simulink model "simpleThermalModel_old"  (R2022a)
settings: Solver=VariableStepAuto  StartTime=0.0  StopTime=36000  RelTol=1e-3
undefined symbols (not defined in the file): param
libraries: fl_lib x53, nesl_utility x15
settings Model: Creator=BrunoMattos  LastModifiedBy=BrunoMattos

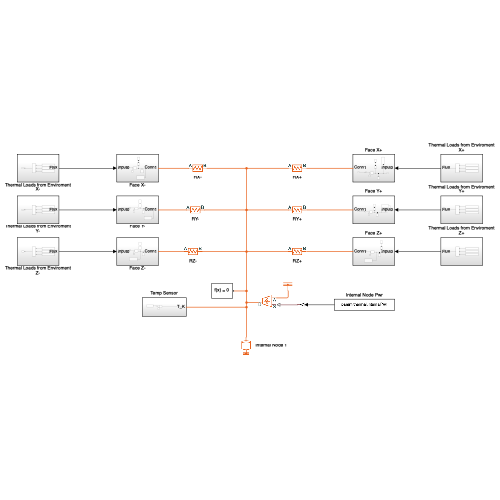
[thumbnail: Simulink's stored preview of the top-level diagram]
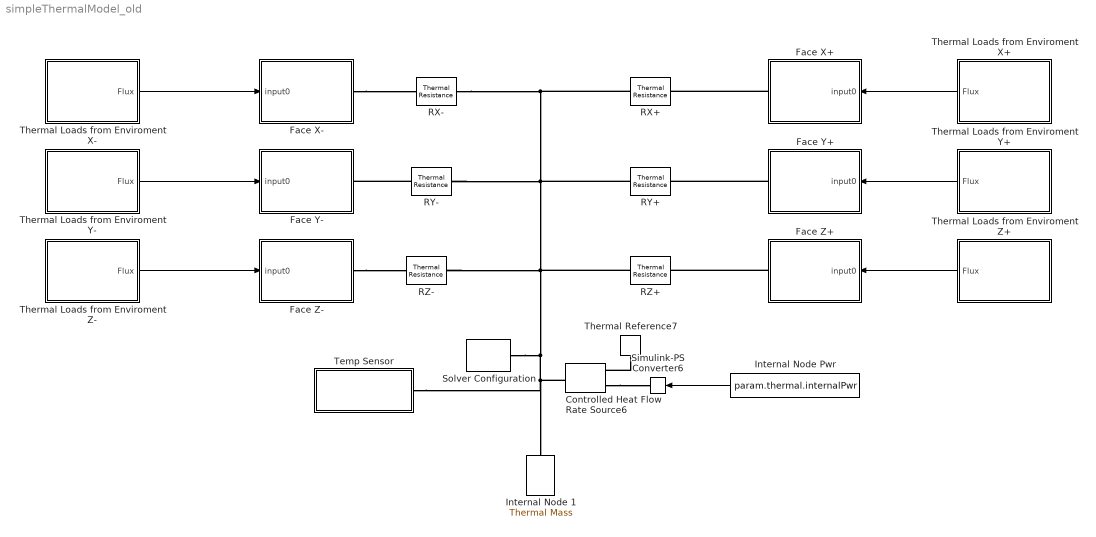
== system simpleThermalModel_old ==
  Controlled Heat Flow Rate Source6 : fl_lib/Thermal/Thermal Sources/Controlled Heat Flow Rate Source
      settings: SourceProductBaseCode=PW,SS,VE
  Face X+ : Subsystem
  Face X- : Subsystem
  Face Y+ : Subsystem
  Face Y- : Subsystem
  Face Z+ : Subsystem
  Face Z- : Subsystem
  Internal Node 1 : fl_lib/Thermal/Thermal Elements/Thermal Mass  mass=param.internalNodeMass(1) kg  sp_heat=param.internalNodeCp(1) J/(K*kg)  T_specify=off  T_priority=High  T=300 K  T_nominal_specify=off  T_nominal_unit=K  T_nominal_value=1  Q_specify=off  Q_priority=None  Q=0 W  Q_nominal_specify=off  Q_nominal_unit=W  Q_nominal_value=1
      settings: SourceProductBaseCode=PW,SS,VE
  Internal Node Pwr : FromWorkspace  VariableName=param.thermal.internalPwr
  RX+ : fl_lib/Thermal/Thermal Elements/Thermal Resistance  resistance=param.resistance(1) K/W  T_specify=off  T_priority=None  T=0 K  T_nominal_specify=off  T_nominal_unit=K  T_nominal_value=1  Q_specify=off  Q_priority=None  Q=0 W  Q_nominal_specify=off  Q_nominal_unit=W  Q_nominal_value=1
      settings: SourceProductBaseCode=PW,SS,VE
  RX- : fl_lib/Thermal/Thermal Elements/Thermal Resistance  resistance=param.resistance(2) K/W  T_specify=off  T_priority=None  T=0 K  T_nominal_specify=off  T_nominal_unit=K  T_nominal_value=1  Q_specify=off  Q_priority=None  Q=0 W  Q_nominal_specify=off  Q_nominal_unit=W  Q_nominal_value=1
      settings: SourceProductBaseCode=PW,SS,VE
  RY+ : fl_lib/Thermal/Thermal Elements/Thermal Resistance  resistance=param.resistance(3) K/W  T_specify=off  T_priority=None  T=0 K  T_nominal_specify=off  T_nominal_unit=K  T_nominal_value=1  Q_specify=off  Q_priority=None  Q=0 W  Q_nominal_specify=off  Q_nominal_unit=W  Q_nominal_value=1
      settings: SourceProductBaseCode=PW,SS,VE
  RY- : fl_lib/Thermal/Thermal Elements/Thermal Resistance  resistance=param.resistance(4) K/W  T_specify=off  T_priority=None  T=0 K  T_nominal_specify=off  T_nominal_unit=K  T_nominal_value=1  Q_specify=off  Q_priority=None  Q=0 W  Q_nominal_specify=off  Q_nominal_unit=W  Q_nominal_value=1
      settings: SourceProductBaseCode=PW,SS,VE
  RZ+ : fl_lib/Thermal/Thermal Elements/Thermal Resistance  resistance=param.resistance(5) K/W  T_specify=off  T_priority=None  T=0 K  T_nominal_specify=off  T_nominal_unit=K  T_nominal_value=1  Q_specify=off  Q_priority=None  Q=0 W  Q_nominal_specify=off  Q_nominal_unit=W  Q_nominal_value=1
      settings: SourceProductBaseCode=PW,SS,VE
  RZ- : fl_lib/Thermal/Thermal Elements/Thermal Resistance  resistance=param.resistance(6) K/W  T_specify=off  T_priority=None  T=0 K  T_nominal_specify=off  T_nominal_unit=K  T_nominal_value=1  Q_specify=off  Q_priority=None  Q=0 W  Q_nominal_specify=off  Q_nominal_unit=W  Q_nominal_value=1
      settings: SourceProductBaseCode=PW,SS,VE
  Simulink-PS Converter6 : nesl_utility/Simulink-PS Converter  PhysicalDomain=network_engine_domain  SubClassName=ps_input  LeftPortType=input  RightPortType=output  PseudoPeriodic=off  Frequencies=[]  NoiseDistribution=none  NoiseParameters=[]  Unit=1  AffineConversion=off  FilteringAndDerivatives=provide  SimscapeFilterOrder=1  InputFilterTimeConstant=0.001  UdotUserProvided=0
      settings: SourceProductBaseCode=SS,PW,VE
  Solver Configuration : nesl_utility/Solver Configuration  PhysicalDomain=network_engine_domain  SubClassName=solver  LeftPortType=input  RightPortType=generic  Tones=[]  Harmonics=[]  SimulateNoise=off  Profile=off  UseLocalSampling=off  EnableSwitchedLinearOptims=on  FrequencyDomain=off  UseCCode=off  RelTol=0.001  AbsTol=0.001  MinStep=1e-09  ToWorkspace=off  RevertToSquareIcSolve=off  NumHomotopyIterations=100  PhasorMode=off  PhasorModeNumHarmonics=1  IndexReductionMethod=DerivativeReplacement  DoDC=off  ResidualTolerance=1e-09  UseLocalSolver=off  LocalSolverChoice=NE_BACKWARD_EULER_ADVANCER  LocalSolverSampleTime=0.001  DoFixedCost=off  MaxNonlinIter=3  MaxModeIter=2  ComputeImpulses=off  ImpulseIterations=2  LinearAlgebra=auto  LinearAlgebraNumThread=0  EquationFormulation=NE_TIME_EF  DelaysMemoryBudget=1024  AutomaticFiltering=on  FilteringTimeConstant=0.001  PartitionStorageMethod=AS_NEEDED  PartitionMemoryBudget=1024  PartitionMethod=ROBUST
      settings: SourceProductBaseCode=SS,PW,VE
  Temp Sensor : Subsystem
  Thermal Loads from Enviroment X+ : Subsystem
  Thermal Loads from Enviroment X- : Subsystem
  Thermal Loads from Enviroment Y+ : Subsystem
  Thermal Loads from Enviroment Y- : Subsystem
  Thermal Loads from Enviroment Z+ : Subsystem
  Thermal Loads from Enviroment Z- : Subsystem
  Thermal Reference7 : fl_lib/Thermal/Thermal Elements/Thermal Reference
      settings: SourceProductBaseCode=PW,SS,VE
  wires:
  Thermal Loads from Enviroment X+/1(Flux) -> Face X+/1(input0)
  Thermal Loads from Enviroment Y+/1(Flux) -> Face Y+/1(input0)
  Thermal Loads from Enviroment Z+/1(Flux) -> Face Z+/1(input0)
  Thermal Loads from Enviroment X-/1(Flux) -> Face X-/1(input0)
  Thermal Loads from Enviroment Y-/1(Flux) -> Face Y-/1(input0)
  Thermal Loads from Enviroment Z-/1(Flux) -> Face Z-/1(input0)
  Internal Node Pwr/1 -> Simulink-PS Converter6/1
  connections:
  RX+/LConn1 -- RX-/RConn1 -- Temp Sensor/LConn1 -- Internal Node 1/LConn1 -- Controlled Heat Flow Rate Source6/LConn1 -- Solver Configuration/RConn1 -- RZ-/RConn1 -- RZ+/LConn1 -- RY-/RConn1 -- RY+/LConn1
  Thermal Reference7/LConn1 -- Controlled Heat Flow Rate Source6/RConn2
  Controlled Heat Flow Rate Source6/RConn1 -- Simulink-PS Converter6/RConn1
  Face X-/RConn1 -- RX-/LConn1
  RY-/LConn1 -- Face Y-/RConn1
  Face Z-/RConn1 -- RZ-/LConn1
  Face X+/RConn1 -- RX+/RConn1
  Face Y+/RConn1 -- RY+/RConn1
  Face Z+/RConn1 -- RZ+/RConn1

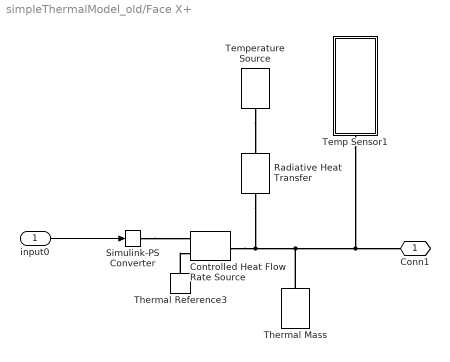
== system simpleThermalModel_old/Face X+ ==
  input0 : Inport
  Controlled Heat Flow Rate Source : fl_lib/Thermal/Thermal Sources/Controlled Heat Flow Rate Source
      settings: SourceProductBaseCode=PW,SS,VE
  Radiative Heat Transfer : fl_lib/Thermal/Thermal Elements/Radiative Heat Transfer  area=param.facesArea(1) m^2  rad_tr_coeff=param.krad(1) W/(K^4*m^2)  T_specify=off  T_priority=None  T=0 K  T_nominal_specify=off  T_nominal_unit=K  T_nominal_value=1  Q_specify=off  Q_priority=None  Q=0 W  Q_nominal_specify=off  Q_nominal_unit=W  Q_nominal_value=1
      settings: SourceProductBaseCode=PW,SS,VE  InternalSimscapePortConfiguration="{\"Bottom\":[],\"Left\":[{\"id\":\"A\",\"label\":\"A\",\"type\":\"foundation.thermal.thermal\"}],\"Right\":[{\"id\":\"B\",\"label\":\"B\",\"type\":\"foundation.thermal.thermal\"}],\"Top\":[]}"
  Simulink-PS Converter : nesl_utility/Simulink-PS Converter  PhysicalDomain=network_engine_domain  SubClassName=ps_input  LeftPortType=input  RightPortType=output  PseudoPeriodic=off  Frequencies=[]  NoiseDistribution=none  NoiseParameters=[]  Unit=1  AffineConversion=off  FilteringAndDerivatives=provide  SimscapeFilterOrder=1  InputFilterTimeConstant=0.001  UdotUserProvided=0
      settings: SourceProductBaseCode=SS,PW,VE
  Temp Sensor1 : Subsystem
  Temperature Source : fl_lib/Thermal/Thermal Sources/Temperature Source  temperature=7 K
      settings: SourceProductBaseCode=PW,SS,VE
  Thermal Mass : fl_lib/Thermal/Thermal Elements/Thermal Mass  mass=param.facesMass(1) kg  sp_heat=param.facesCp(1) J/(K*kg)  T_specify=off  T_priority=High  T=300 K  T_nominal_specify=off  T_nominal_unit=K  T_nominal_value=1  Q_specify=off  Q_priority=None  Q=0 W  Q_nominal_specify=off  Q_nominal_unit=W  Q_nominal_value=1
      settings: SourceProductBaseCode=PW,SS,VE
  Thermal Reference3 : fl_lib/Thermal/Thermal Elements/Thermal Reference
      settings: SourceProductBaseCode=PW,SS,VE
  Conn1 : PMIOPort  Side=Right
  wires:
  input0/1 -> Simulink-PS Converter/1
  connections:
  Simulink-PS Converter/RConn1 -- Controlled Heat Flow Rate Source/RConn1
  Thermal Reference3/LConn1 -- Controlled Heat Flow Rate Source/RConn2
  Temperature Source/LConn1 -- Radiative Heat Transfer/RConn1
  Radiative Heat Transfer/LConn1 -- Controlled Heat Flow Rate Source/LConn1 -- Thermal Mass/LConn1 -- Temp Sensor1/LConn1 -- Conn1/RConn1

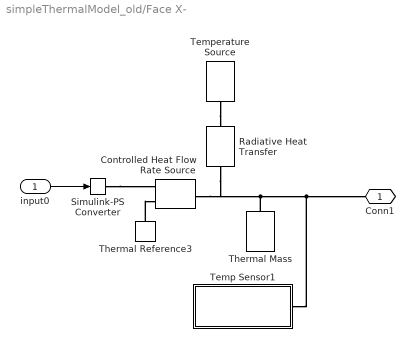
== system simpleThermalModel_old/Face X- ==
  input0 : Inport
  Controlled Heat Flow Rate Source : fl_lib/Thermal/Thermal Sources/Controlled Heat Flow Rate Source
      settings: SourceProductBaseCode=PW,SS,VE
  Radiative Heat Transfer : fl_lib/Thermal/Thermal Elements/Radiative Heat Transfer  area=param.facesArea(2) m^2  rad_tr_coeff=param.krad(2) W/(K^4*m^2)  T_specify=off  T_priority=None  T=0 K  T_nominal_specify=off  T_nominal_unit=K  T_nominal_value=1  Q_specify=off  Q_priority=None  Q=0 W  Q_nominal_specify=off  Q_nominal_unit=W  Q_nominal_value=1
      settings: SourceProductBaseCode=PW,SS,VE  InternalSimscapePortConfiguration="{\"Bottom\":[],\"Left\":[{\"id\":\"A\",\"label\":\"A\",\"type\":\"foundation.thermal.thermal\"}],\"Right\":[{\"id\":\"B\",\"label\":\"B\",\"type\":\"foundation.thermal.thermal\"}],\"Top\":[]}"
  Simulink-PS Converter : nesl_utility/Simulink-PS Converter  PhysicalDomain=network_engine_domain  SubClassName=ps_input  LeftPortType=input  RightPortType=output  PseudoPeriodic=off  Frequencies=[]  NoiseDistribution=none  NoiseParameters=[]  Unit=1  AffineConversion=off  FilteringAndDerivatives=provide  SimscapeFilterOrder=1  InputFilterTimeConstant=0.001  UdotUserProvided=0
      settings: SourceProductBaseCode=SS,PW,VE
  Temp Sensor1 : Subsystem
  Temperature Source : fl_lib/Thermal/Thermal Sources/Temperature Source  temperature=7 K
      settings: SourceProductBaseCode=PW,SS,VE
  Thermal Mass : fl_lib/Thermal/Thermal Elements/Thermal Mass  mass=param.facesMass(2) kg  sp_heat=param.facesCp(2) J/(K*kg)  T_specify=off  T_priority=High  T=300 K  T_nominal_specify=off  T_nominal_unit=K  T_nominal_value=1  Q_specify=off  Q_priority=None  Q=0 W  Q_nominal_specify=off  Q_nominal_unit=W  Q_nominal_value=1
      settings: SourceProductBaseCode=PW,SS,VE
  Thermal Reference3 : fl_lib/Thermal/Thermal Elements/Thermal Reference
      settings: SourceProductBaseCode=PW,SS,VE
  Conn1 : PMIOPort  Side=Right
  wires:
  input0/1 -> Simulink-PS Converter/1
  connections:
  Simulink-PS Converter/RConn1 -- Controlled Heat Flow Rate Source/RConn1
  Thermal Reference3/LConn1 -- Controlled Heat Flow Rate Source/RConn2
  Temperature Source/LConn1 -- Radiative Heat Transfer/RConn1
  Thermal Mass/LConn1 -- Temp Sensor1/LConn1 -- Conn1/RConn1 -- Radiative Heat Transfer/LConn1 -- Controlled Heat Flow Rate Source/LConn1

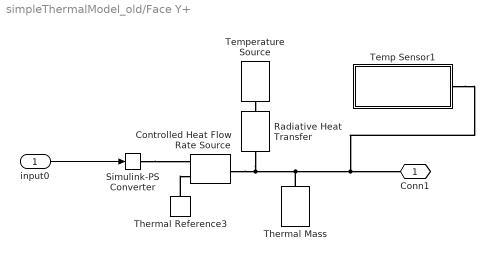
== system simpleThermalModel_old/Face Y+ ==
  input0 : Inport
  Controlled Heat Flow Rate Source : fl_lib/Thermal/Thermal Sources/Controlled Heat Flow Rate Source
      settings: SourceProductBaseCode=PW,SS,VE
  Radiative Heat Transfer : fl_lib/Thermal/Thermal Elements/Radiative Heat Transfer  area=param.facesArea(3) m^2  rad_tr_coeff=param.krad(3) W/(K^4*m^2)  T_specify=off  T_priority=None  T=0 K  T_nominal_specify=off  T_nominal_unit=K  T_nominal_value=1  Q_specify=off  Q_priority=None  Q=0 W  Q_nominal_specify=off  Q_nominal_unit=W  Q_nominal_value=1
      settings: SourceProductBaseCode=PW,SS,VE  InternalSimscapePortConfiguration="{\"Bottom\":[],\"Left\":[{\"id\":\"A\",\"label\":\"A\",\"type\":\"foundation.thermal.thermal\"}],\"Right\":[{\"id\":\"B\",\"label\":\"B\",\"type\":\"foundation.thermal.thermal\"}],\"Top\":[]}"
  Simulink-PS Converter : nesl_utility/Simulink-PS Converter  PhysicalDomain=network_engine_domain  SubClassName=ps_input  LeftPortType=input  RightPortType=output  PseudoPeriodic=off  Frequencies=[]  NoiseDistribution=none  NoiseParameters=[]  Unit=1  AffineConversion=off  FilteringAndDerivatives=provide  SimscapeFilterOrder=1  InputFilterTimeConstant=0.001  UdotUserProvided=0
      settings: SourceProductBaseCode=SS,PW,VE
  Temp Sensor1 : Subsystem
  Temperature Source : fl_lib/Thermal/Thermal Sources/Temperature Source  temperature=7 K
      settings: SourceProductBaseCode=PW,SS,VE
  Thermal Mass : fl_lib/Thermal/Thermal Elements/Thermal Mass  mass=param.facesMass(3) kg  sp_heat=param.facesCp(3) J/(K*kg)  T_specify=off  T_priority=High  T=300 K  T_nominal_specify=off  T_nominal_unit=K  T_nominal_value=1  Q_specify=off  Q_priority=None  Q=0 W  Q_nominal_specify=off  Q_nominal_unit=W  Q_nominal_value=1
      settings: SourceProductBaseCode=PW,SS,VE
  Thermal Reference3 : fl_lib/Thermal/Thermal Elements/Thermal Reference
      settings: SourceProductBaseCode=PW,SS,VE
  Conn1 : PMIOPort  Side=Right
  wires:
  input0/1 -> Simulink-PS Converter/1
  connections:
  Simulink-PS Converter/RConn1 -- Controlled Heat Flow Rate Source/RConn1
  Thermal Reference3/LConn1 -- Controlled Heat Flow Rate Source/RConn2
  Temperature Source/LConn1 -- Radiative Heat Transfer/RConn1
  Radiative Heat Transfer/LConn1 -- Controlled Heat Flow Rate Source/LConn1 -- Thermal Mass/LConn1 -- Temp Sensor1/LConn1 -- Conn1/RConn1

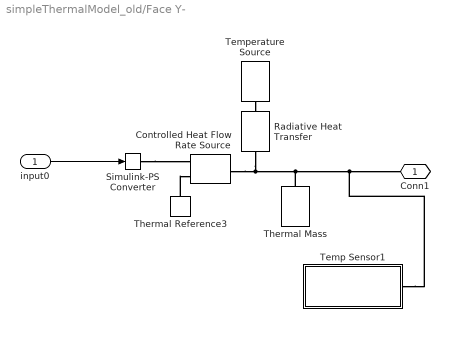
== system simpleThermalModel_old/Face Y- ==
  input0 : Inport
  Controlled Heat Flow Rate Source : fl_lib/Thermal/Thermal Sources/Controlled Heat Flow Rate Source
      settings: SourceProductBaseCode=PW,SS,VE
  Radiative Heat Transfer : fl_lib/Thermal/Thermal Elements/Radiative Heat Transfer  area=param.facesArea(4) m^2  rad_tr_coeff=param.krad(4) W/(K^4*m^2)  T_specify=off  T_priority=None  T=0 K  T_nominal_specify=off  T_nominal_unit=K  T_nominal_value=1  Q_specify=off  Q_priority=None  Q=0 W  Q_nominal_specify=off  Q_nominal_unit=W  Q_nominal_value=1
      settings: SourceProductBaseCode=PW,SS,VE  InternalSimscapePortConfiguration="{\"Bottom\":[],\"Left\":[{\"id\":\"A\",\"label\":\"A\",\"type\":\"foundation.thermal.thermal\"}],\"Right\":[{\"id\":\"B\",\"label\":\"B\",\"type\":\"foundation.thermal.thermal\"}],\"Top\":[]}"
  Simulink-PS Converter : nesl_utility/Simulink-PS Converter  PhysicalDomain=network_engine_domain  SubClassName=ps_input  LeftPortType=input  RightPortType=output  PseudoPeriodic=off  Frequencies=[]  NoiseDistribution=none  NoiseParameters=[]  Unit=1  AffineConversion=off  FilteringAndDerivatives=provide  SimscapeFilterOrder=1  InputFilterTimeConstant=0.001  UdotUserProvided=0
      settings: SourceProductBaseCode=SS,PW,VE
  Temp Sensor1 : Subsystem
  Temperature Source : fl_lib/Thermal/Thermal Sources/Temperature Source  temperature=7 K
      settings: SourceProductBaseCode=PW,SS,VE
  Thermal Mass : fl_lib/Thermal/Thermal Elements/Thermal Mass  mass=param.facesMass(4) kg  sp_heat=param.facesCp(4) J/(K*kg)  T_specify=off  T_priority=High  T=300 K  T_nominal_specify=off  T_nominal_unit=K  T_nominal_value=1  Q_specify=off  Q_priority=None  Q=0 W  Q_nominal_specify=off  Q_nominal_unit=W  Q_nominal_value=1
      settings: SourceProductBaseCode=PW,SS,VE
  Thermal Reference3 : fl_lib/Thermal/Thermal Elements/Thermal Reference
      settings: SourceProductBaseCode=PW,SS,VE
  Conn1 : PMIOPort  Side=Right
  wires:
  input0/1 -> Simulink-PS Converter/1
  connections:
  Simulink-PS Converter/RConn1 -- Controlled Heat Flow Rate Source/RConn1
  Thermal Reference3/LConn1 -- Controlled Heat Flow Rate Source/RConn2
  Temperature Source/LConn1 -- Radiative Heat Transfer/RConn1
  Radiative Heat Transfer/LConn1 -- Controlled Heat Flow Rate Source/LConn1 -- Thermal Mass/LConn1 -- Temp Sensor1/LConn1 -- Conn1/RConn1

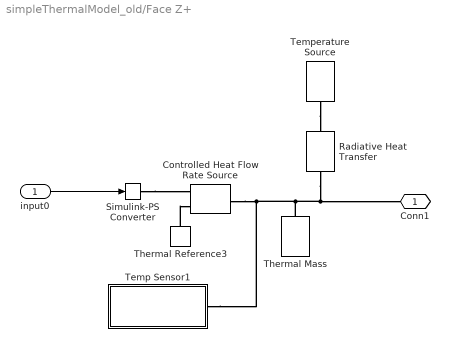
== system simpleThermalModel_old/Face Z+ ==
  input0 : Inport
  Controlled Heat Flow Rate Source : fl_lib/Thermal/Thermal Sources/Controlled Heat Flow Rate Source
      settings: SourceProductBaseCode=PW,SS,VE
  Radiative Heat Transfer : fl_lib/Thermal/Thermal Elements/Radiative Heat Transfer  area=param.facesArea(5) m^2  rad_tr_coeff=param.krad(5) W/(K^4*m^2)  T_specify=off  T_priority=None  T=0 K  T_nominal_specify=off  T_nominal_unit=K  T_nominal_value=1  Q_specify=off  Q_priority=None  Q=0 W  Q_nominal_specify=off  Q_nominal_unit=W  Q_nominal_value=1
      settings: SourceProductBaseCode=PW,SS,VE  InternalSimscapePortConfiguration="{\"Bottom\":[],\"Left\":[{\"id\":\"A\",\"label\":\"A\",\"type\":\"foundation.thermal.thermal\"}],\"Right\":[{\"id\":\"B\",\"label\":\"B\",\"type\":\"foundation.thermal.thermal\"}],\"Top\":[]}"
  Simulink-PS Converter : nesl_utility/Simulink-PS Converter  PhysicalDomain=network_engine_domain  SubClassName=ps_input  LeftPortType=input  RightPortType=output  PseudoPeriodic=off  Frequencies=[]  NoiseDistribution=none  NoiseParameters=[]  Unit=1  AffineConversion=off  FilteringAndDerivatives=provide  SimscapeFilterOrder=1  InputFilterTimeConstant=0.001  UdotUserProvided=0
      settings: SourceProductBaseCode=SS,PW,VE
  Temp Sensor1 : Subsystem
  Temperature Source : fl_lib/Thermal/Thermal Sources/Temperature Source  temperature=7 K
      settings: SourceProductBaseCode=PW,SS,VE
  Thermal Mass : fl_lib/Thermal/Thermal Elements/Thermal Mass  mass=param.facesMass(5) kg  sp_heat=param.facesCp(5) J/(K*kg)  T_specify=off  T_priority=High  T=300 K  T_nominal_specify=off  T_nominal_unit=K  T_nominal_value=1  Q_specify=off  Q_priority=None  Q=0 W  Q_nominal_specify=off  Q_nominal_unit=W  Q_nominal_value=1
      settings: SourceProductBaseCode=PW,SS,VE
  Thermal Reference3 : fl_lib/Thermal/Thermal Elements/Thermal Reference
      settings: SourceProductBaseCode=PW,SS,VE
  Conn1 : PMIOPort  Side=Right
  wires:
  input0/1 -> Simulink-PS Converter/1
  connections:
  Simulink-PS Converter/RConn1 -- Controlled Heat Flow Rate Source/RConn1
  Thermal Reference3/LConn1 -- Controlled Heat Flow Rate Source/RConn2
  Temperature Source/LConn1 -- Radiative Heat Transfer/RConn1
  Radiative Heat Transfer/LConn1 -- Controlled Heat Flow Rate Source/LConn1 -- Temp Sensor1/LConn1 -- Thermal Mass/LConn1 -- Conn1/RConn1

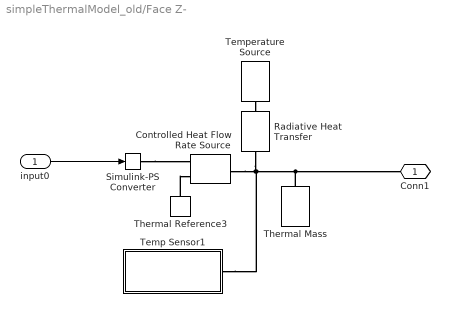
== system simpleThermalModel_old/Face Z- ==
  input0 : Inport
  Controlled Heat Flow Rate Source : fl_lib/Thermal/Thermal Sources/Controlled Heat Flow Rate Source
      settings: SourceProductBaseCode=PW,SS,VE
  Radiative Heat Transfer : fl_lib/Thermal/Thermal Elements/Radiative Heat Transfer  area=param.facesArea(6) m^2  rad_tr_coeff=param.krad(6) W/(K^4*m^2)  T_specify=off  T_priority=None  T=0 K  T_nominal_specify=off  T_nominal_unit=K  T_nominal_value=1  Q_specify=off  Q_priority=None  Q=0 W  Q_nominal_specify=off  Q_nominal_unit=W  Q_nominal_value=1
      settings: SourceProductBaseCode=PW,SS,VE  InternalSimscapePortConfiguration="{\"Bottom\":[],\"Left\":[{\"id\":\"A\",\"label\":\"A\",\"type\":\"foundation.thermal.thermal\"}],\"Right\":[{\"id\":\"B\",\"label\":\"B\",\"type\":\"foundation.thermal.thermal\"}],\"Top\":[]}"
  Simulink-PS Converter : nesl_utility/Simulink-PS Converter  PhysicalDomain=network_engine_domain  SubClassName=ps_input  LeftPortType=input  RightPortType=output  PseudoPeriodic=off  Frequencies=[]  NoiseDistribution=none  NoiseParameters=[]  Unit=1  AffineConversion=off  FilteringAndDerivatives=provide  SimscapeFilterOrder=1  InputFilterTimeConstant=0.001  UdotUserProvided=0
      settings: SourceProductBaseCode=SS,PW,VE
  Temp Sensor1 : Subsystem
  Temperature Source : fl_lib/Thermal/Thermal Sources/Temperature Source  temperature=7 K
      settings: SourceProductBaseCode=PW,SS,VE
  Thermal Mass : fl_lib/Thermal/Thermal Elements/Thermal Mass  mass=param.facesMass(6) kg  sp_heat=param.facesCp(6) J/(K*kg)  T_specify=off  T_priority=High  T=300 K  T_nominal_specify=off  T_nominal_unit=K  T_nominal_value=1  Q_specify=off  Q_priority=None  Q=0 W  Q_nominal_specify=off  Q_nominal_unit=W  Q_nominal_value=1
      settings: SourceProductBaseCode=PW,SS,VE
  Thermal Reference3 : fl_lib/Thermal/Thermal Elements/Thermal Reference
      settings: SourceProductBaseCode=PW,SS,VE
  Conn1 : PMIOPort  Side=Right
  wires:
  input0/1 -> Simulink-PS Converter/1
  connections:
  Simulink-PS Converter/RConn1 -- Controlled Heat Flow Rate Source/RConn1
  Thermal Reference3/LConn1 -- Controlled Heat Flow Rate Source/RConn2
  Temperature Source/LConn1 -- Radiative Heat Transfer/RConn1
  Radiative Heat Transfer/LConn1 -- Controlled Heat Flow Rate Source/LConn1 -- Thermal Mass/LConn1 -- Conn1/RConn1 -- Temp Sensor1/LConn1

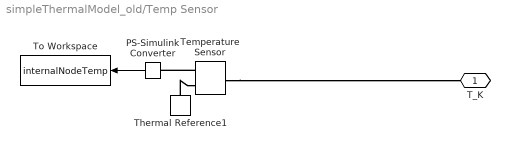
== system simpleThermalModel_old/Temp Sensor ==
  PS-Simulink Converter : nesl_utility/PS-Simulink Converter  PhysicalDomain=network_engine_domain  SubClassName=ps_output  LeftPortType=input  RightPortType=output  PseudoPeriodic=off  Frequencies=[]  VectorFormat=inherit  Unit=inherit  AffineConversion=off
      settings: SourceProductBaseCode=SS,PW,VE
  Temperature Sensor : fl_lib/Thermal/Thermal Sensors/Temperature Sensor
      settings: SourceProductBaseCode=PW,SS,VE
  Thermal Reference1 : fl_lib/Thermal/Thermal Elements/Thermal Reference
      settings: SourceProductBaseCode=PW,SS,VE
  To Workspace : ToWorkspace  VariableName=internalNodeTemp  SaveFormat=Timeseries  SampleTime=-1
  T_K : PMIOPort  Side=Left
  wires:
  PS-Simulink Converter/1 -> To Workspace/1
  connections:
  Temperature Sensor/LConn1 -- T_K/RConn1
  Temperature Sensor/RConn2 -- PS-Simulink Converter/LConn1
  Thermal Reference1/LConn1 -- Temperature Sensor/RConn1

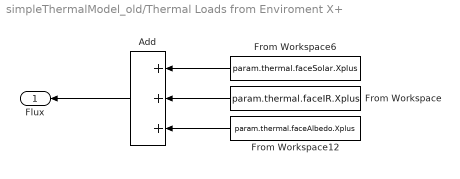
== system simpleThermalModel_old/Thermal Loads from Enviroment X+ ==
  Add : Sum  Inputs=+++
  From Workspace : FromWorkspace  VariableName=param.thermal.faceIR.Xplus
  From Workspace12 : FromWorkspace  VariableName=param.thermal.faceAlbedo.Xplus
  From Workspace6 : FromWorkspace  VariableName=param.thermal.faceSolar.Xplus
  Flux : Outport
  wires:
  From Workspace12/1 -> Add/3
  From Workspace6/1 -> Add/1
  Add/1 -> Flux/1
  From Workspace/1 -> Add/2

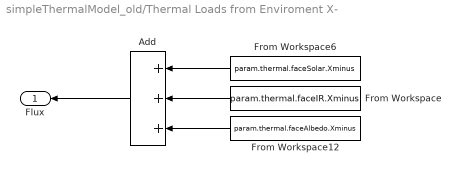
== system simpleThermalModel_old/Thermal Loads from Enviroment X- ==
  Add : Sum  Inputs=+++
  From Workspace : FromWorkspace  VariableName=param.thermal.faceIR.Xminus
  From Workspace12 : FromWorkspace  VariableName=param.thermal.faceAlbedo.Xminus
  From Workspace6 : FromWorkspace  VariableName=param.thermal.faceSolar.Xminus
  Flux : Outport
  wires:
  From Workspace12/1 -> Add/3
  From Workspace6/1 -> Add/1
  Add/1 -> Flux/1
  From Workspace/1 -> Add/2

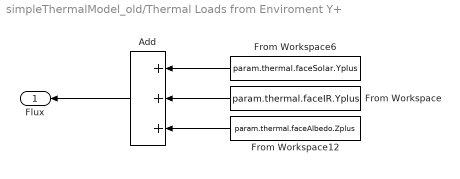
== system simpleThermalModel_old/Thermal Loads from Enviroment Y+ ==
  Add : Sum  Inputs=+++
  From Workspace : FromWorkspace  VariableName=param.thermal.faceIR.Yplus
  From Workspace12 : FromWorkspace  VariableName=param.thermal.faceAlbedo.Zplus
  From Workspace6 : FromWorkspace  VariableName=param.thermal.faceSolar.Yplus
  Flux : Outport
  wires:
  From Workspace12/1 -> Add/3
  From Workspace6/1 -> Add/1
  Add/1 -> Flux/1
  From Workspace/1 -> Add/2

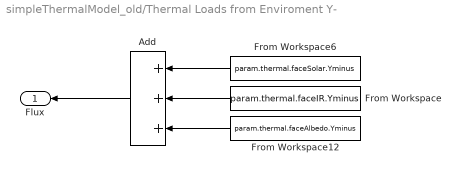
== system simpleThermalModel_old/Thermal Loads from Enviroment Y- ==
  Add : Sum  Inputs=+++
  From Workspace : FromWorkspace  VariableName=param.thermal.faceIR.Yminus
  From Workspace12 : FromWorkspace  VariableName=param.thermal.faceAlbedo.Yminus
  From Workspace6 : FromWorkspace  VariableName=param.thermal.faceSolar.Yminus
  Flux : Outport
  wires:
  From Workspace12/1 -> Add/3
  From Workspace6/1 -> Add/1
  Add/1 -> Flux/1
  From Workspace/1 -> Add/2

== system simpleThermalModel_old/Thermal Loads from Enviroment Z+ ==
  Add : Sum  Inputs=+++
  From Workspace : FromWorkspace  VariableName=param.thermal.faceIR.Zplus
  From Workspace12 : FromWorkspace  VariableName=param.thermal.faceAlbedo.Zplus
  From Workspace6 : FromWorkspace  VariableName=param.thermal.faceSolar.Zplus
  Flux : Outport
  wires:
  From Workspace12/1 -> Add/3
  From Workspace6/1 -> Add/1
  Add/1 -> Flux/1
  From Workspace/1 -> Add/2

== system simpleThermalModel_old/Thermal Loads from Enviroment Z- ==
  Add : Sum  Inputs=+++
  From Workspace : FromWorkspace  VariableName=param.thermal.faceIR.Zminus
  From Workspace12 : FromWorkspace  VariableName=param.thermal.faceAlbedo.Zminus
  From Workspace6 : FromWorkspace  VariableName=param.thermal.faceSolar.Zminus
  Flux : Outport
  wires:
  From Workspace12/1 -> Add/3
  From Workspace6/1 -> Add/1
  Add/1 -> Flux/1
  From Workspace/1 -> Add/2

== system simpleThermalModel_old/Face X+/Temp Sensor1 ==
  PS-Simulink Converter : nesl_utility/PS-Simulink Converter  PhysicalDomain=network_engine_domain  SubClassName=ps_output  LeftPortType=input  RightPortType=output  PseudoPeriodic=off  Frequencies=[]  VectorFormat=inherit  Unit=inherit  AffineConversion=off
      settings: SourceProductBaseCode=SS,PW,VE
  Temperature Sensor : fl_lib/Thermal/Thermal Sensors/Temperature Sensor
      settings: SourceProductBaseCode=PW,SS,VE
  Thermal Reference1 : fl_lib/Thermal/Thermal Elements/Thermal Reference
      settings: SourceProductBaseCode=PW,SS,VE
  To Workspace : ToWorkspace  VariableName=XplusTemp  SaveFormat=Timeseries  SampleTime=-1
  T_K : PMIOPort  Side=Left
  wires:
  PS-Simulink Converter/1 -> To Workspace/1
  connections:
  Temperature Sensor/LConn1 -- T_K/RConn1
  Temperature Sensor/RConn2 -- PS-Simulink Converter/LConn1
  Thermal Reference1/LConn1 -- Temperature Sensor/RConn1

== system simpleThermalModel_old/Face X-/Temp Sensor1 ==
  PS-Simulink Converter : nesl_utility/PS-Simulink Converter  PhysicalDomain=network_engine_domain  SubClassName=ps_output  LeftPortType=input  RightPortType=output  PseudoPeriodic=off  Frequencies=[]  VectorFormat=inherit  Unit=inherit  AffineConversion=off
      settings: SourceProductBaseCode=SS,PW,VE
  Temperature Sensor : fl_lib/Thermal/Thermal Sensors/Temperature Sensor
      settings: SourceProductBaseCode=PW,SS,VE
  Thermal Reference1 : fl_lib/Thermal/Thermal Elements/Thermal Reference
      settings: SourceProductBaseCode=PW,SS,VE
  To Workspace : ToWorkspace  VariableName=XminusTemp  SaveFormat=Timeseries  SampleTime=-1
  T_K : PMIOPort  Side=Left
  wires:
  PS-Simulink Converter/1 -> To Workspace/1
  connections:
  Temperature Sensor/LConn1 -- T_K/RConn1
  Temperature Sensor/RConn2 -- PS-Simulink Converter/LConn1
  Thermal Reference1/LConn1 -- Temperature Sensor/RConn1

== system simpleThermalModel_old/Face Y+/Temp Sensor1 ==
  PS-Simulink Converter : nesl_utility/PS-Simulink Converter  PhysicalDomain=network_engine_domain  SubClassName=ps_output  LeftPortType=input  RightPortType=output  PseudoPeriodic=off  Frequencies=[]  VectorFormat=inherit  Unit=inherit  AffineConversion=off
      settings: SourceProductBaseCode=SS,PW,VE
  Temperature Sensor : fl_lib/Thermal/Thermal Sensors/Temperature Sensor
      settings: SourceProductBaseCode=PW,SS,VE
  Thermal Reference1 : fl_lib/Thermal/Thermal Elements/Thermal Reference
      settings: SourceProductBaseCode=PW,SS,VE
  To Workspace : ToWorkspace  VariableName=YplusTemp  SaveFormat=Timeseries  SampleTime=-1
  T_K : PMIOPort  Side=Left
  wires:
  PS-Simulink Converter/1 -> To Workspace/1
  connections:
  Temperature Sensor/LConn1 -- T_K/RConn1
  Temperature Sensor/RConn2 -- PS-Simulink Converter/LConn1
  Thermal Reference1/LConn1 -- Temperature Sensor/RConn1

== system simpleThermalModel_old/Face Y-/Temp Sensor1 ==
  PS-Simulink Converter : nesl_utility/PS-Simulink Converter  PhysicalDomain=network_engine_domain  SubClassName=ps_output  LeftPortType=input  RightPortType=output  PseudoPeriodic=off  Frequencies=[]  VectorFormat=inherit  Unit=inherit  AffineConversion=off
      settings: SourceProductBaseCode=SS,PW,VE
  Temperature Sensor : fl_lib/Thermal/Thermal Sensors/Temperature Sensor
      settings: SourceProductBaseCode=PW,SS,VE
  Thermal Reference1 : fl_lib/Thermal/Thermal Elements/Thermal Reference
      settings: SourceProductBaseCode=PW,SS,VE
  To Workspace : ToWorkspace  VariableName=YminusTemp  SaveFormat=Timeseries  SampleTime=-1
  T_K : PMIOPort  Side=Left
  wires:
  PS-Simulink Converter/1 -> To Workspace/1
  connections:
  Temperature Sensor/LConn1 -- T_K/RConn1
  Temperature Sensor/RConn2 -- PS-Simulink Converter/LConn1
  Thermal Reference1/LConn1 -- Temperature Sensor/RConn1

== system simpleThermalModel_old/Face Z+/Temp Sensor1 ==
  PS-Simulink Converter : nesl_utility/PS-Simulink Converter  PhysicalDomain=network_engine_domain  SubClassName=ps_output  LeftPortType=input  RightPortType=output  PseudoPeriodic=off  Frequencies=[]  VectorFormat=inherit  Unit=inherit  AffineConversion=off
      settings: SourceProductBaseCode=SS,PW,VE
  Temperature Sensor : fl_lib/Thermal/Thermal Sensors/Temperature Sensor
      settings: SourceProductBaseCode=PW,SS,VE
  Thermal Reference1 : fl_lib/Thermal/Thermal Elements/Thermal Reference
      settings: SourceProductBaseCode=PW,SS,VE
  To Workspace : ToWorkspace  VariableName=ZplusTemp  SaveFormat=Timeseries  SampleTime=-1
  T_K : PMIOPort  Side=Left
  wires:
  PS-Simulink Converter/1 -> To Workspace/1
  connections:
  Temperature Sensor/LConn1 -- T_K/RConn1
  Temperature Sensor/RConn2 -- PS-Simulink Converter/LConn1
  Thermal Reference1/LConn1 -- Temperature Sensor/RConn1

== system simpleThermalModel_old/Face Z-/Temp Sensor1 ==
  PS-Simulink Converter : nesl_utility/PS-Simulink Converter  PhysicalDomain=network_engine_domain  SubClassName=ps_output  LeftPortType=input  RightPortType=output  PseudoPeriodic=off  Frequencies=[]  VectorFormat=inherit  Unit=inherit  AffineConversion=off
      settings: SourceProductBaseCode=SS,PW,VE
  Temperature Sensor : fl_lib/Thermal/Thermal Sensors/Temperature Sensor
      settings: SourceProductBaseCode=PW,SS,VE
  Thermal Reference1 : fl_lib/Thermal/Thermal Elements/Thermal Reference
      settings: SourceProductBaseCode=PW,SS,VE
  To Workspace : ToWorkspace  VariableName=ZminusTemp  SaveFormat=Timeseries  SampleTime=-1
  T_K : PMIOPort  Side=Left
  wires:
  PS-Simulink Converter/1 -> To Workspace/1
  connections:
  Temperature Sensor/LConn1 -- T_K/RConn1
  Temperature Sensor/RConn2 -- PS-Simulink Converter/LConn1
  Thermal Reference1/LConn1 -- Temperature Sensor/RConn1
